simulink model "brushproportionelF"  (R2021a)
settings: Solver=ode45  StartTime=0.0  StopTime=2.0  RelTol=1e-3  EnableMultiTasking=on
libraries: spsIGBTDiodeLib x6, simulink x3, electricdrivelib x1, spsDCVoltageSourceLib x1, spspowerguiLib x1
settings Model: Creator=hp  LastModifiedBy=HP
settings SolverCC: AlgebraicLoopSolver=TrustRegion
settings DataIOCC: LimitDataPoints=on  SaveFormat=Array  ReturnWorkspaceOutputs=off
settings OptimizationCC: LifeSpan=inf
settings DebuggingCC: UnderspecifiedInitializationDetection=Classic  MergeDetectMultiDrivingBlocksExec=none  SolverPrmCheckMsg=warning  StateNameClashWarn=warning  SFUnexpectedBacktrackingDiag=warning  SFNoUnconditionalDefaultTransitionDiag=warning  SFExecutionAtInitializationDiag=none  SFMachineParentedDataDiag=warning  ArithmeticOperatorsInVariantConditions=warning
settings HardwareCC: ProdBitPerPointer=32  ProdBitPerSizeT=32  ProdBitPerPtrDiffT=32  ProdLargestAtomicFloat=None  ProdIntDivRoundTo=Undefined  ProdEndianess=Unspecified  ProdWordSize=32  ProdHWDeviceType=32-bit Generic
settings ModelReferenceCC: PropagateSignalLabelsOutOfModel=off
settings SFSimCC: SimUseLocalCustomCode=off  CustomCodeUndefinedFunction=UseInterfaceOnly
settings RTWCC: RTWUseLocalCustomCode=off
settings CodeAppCC: StateflowObjectComments=on
settings GRTTargetCC: TargetLangStandard=C89/C90 (ANSI)
settings ConfigComp: CovMetricSettings=dw  CovSaveCumulativeToWorkspaceVar=on  CovSaveSingleToWorkspaceVar=on  CovExternalEMLEnable=off
settings SimscapeCC: SimscapeNormalizeSystem=off

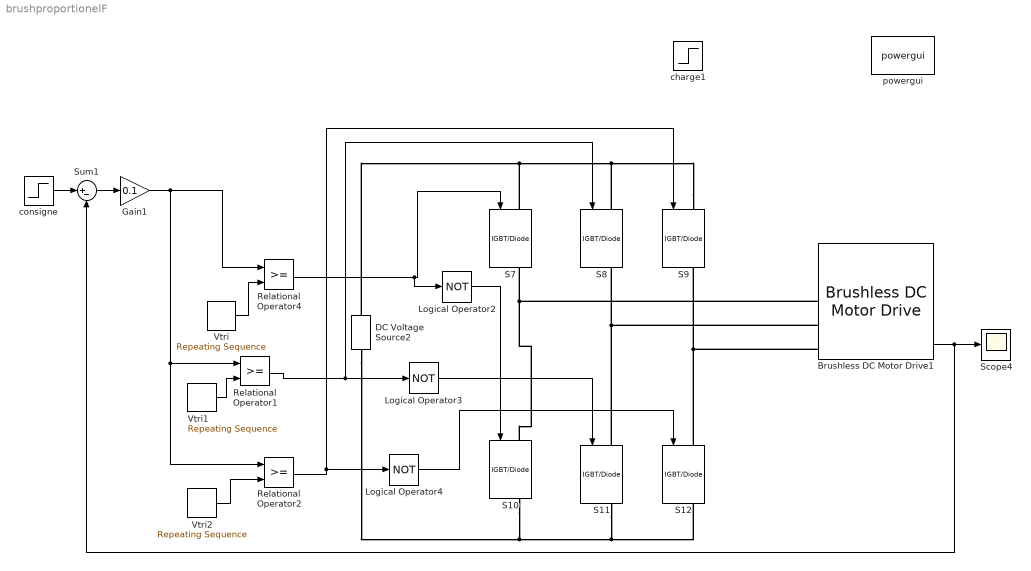
== system brushproportionelF ==
  Brushless DC Motor Drive1 : electricdrivelib/AC drives/Brushless DC Motor Drive  Rs=0.2  Lls=8.5e-3  Flat=120  MachineConstant=Flux linkage established by magnets (V.s)  FluxCst=0.175  VoltageCst=146.6077  TorqueCst=1.4  ia=0  ib=0  J=0.089  Friction=0.005  p=4  wm=0  thetam=0  Rsnb_rec=10e3  Csnb_rec=20e-9  Ron_rec=1e-3  Vf_rec=1.3  cap_bus=2000e-6  Rbrake=8  fbrake=4000  activationVoltage=320  shutdownVoltage=310  deviceType=MOSFET / Diodes  Ron_inv=1e-3  Vf_inv=0.8  Vfd_inv=0.8  Tf=1e-6  Tt=2e-6  Tf_GTO=10e-6  Tt_GTO=20e-6  Rsnb_inv=5000  Csnb_inv=1e-6  regulationType=Speed regulation  Acc=1000  Dec=-1000  kp_sc=5  ki_sc=100  fc_sc=100  Tsc=7*20e-6  Tmin=-17.8  Tmax=17.8  h=0.01  freq_max=20e3  Tvect=20e-6  zeta=0.99  Trd=0.13/5  K1=3000  K2=-49500  baseSampleTime=2e-06  outputBusMode=Multiple output buses  busLabels=off  sensorless=off  MechanicalLoad=Torque Tm  modelDetailLevel=Detailed  driveType=AC7  AverageValue=off
      settings: SourceProductBaseCode=PS
  DC Voltage Source2 : spsDCVoltageSourceLib/DC Voltage Source  Amplitude=240  Measurements=None
  Gain1 : Gain  Gain=0.1
  Logical Operator2 : Logic  Operator=NOT  AllPortsSameDT=off  OutDataTypeStr=boolean
  Logical Operator3 : Logic  Operator=NOT  AllPortsSameDT=off  OutDataTypeStr=boolean
  Logical Operator4 : Logic  Operator=NOT  AllPortsSameDT=off  OutDataTypeStr=boolean
  Relational Operator1 : RelationalOperator  OutDataTypeStr=boolean  RndMeth=Nearest
  Relational Operator2 : RelationalOperator  OutDataTypeStr=boolean  RndMeth=Nearest
  Relational Operator4 : RelationalOperator  OutDataTypeStr=boolean  RndMeth=Nearest
  S{7..12} (6 alike) : spsIGBTDiodeLib/IGBT//Diode  Ron=1e-3  Rs=1e5  Cs=inf  Measurements=on
  Scope4 : Scope
  Sum1 : Sum  Inputs=|+-
  Vtri : simulink/Sources/Repeating Sequence  rep_seq_t=[0 (1/2) 1]*0.001  rep_seq_y="[-1  1 -1] *240"
  Vtri1 : simulink/Sources/Repeating Sequence  rep_seq_t=[0 (1/6) 1]*0.001  rep_seq_y="[-1  1 -1] *240"
  Vtri2 : simulink/Sources/Repeating Sequence  rep_seq_t=[0 (1/3) 1]*0.001  rep_seq_y="[-1  1 -1] *240"
  charge1 : Step  Time=0.1  After=0.1  SampleTime=0
  consigne : Step  Time=0  After=150  SampleTime=0
  powergui : spspowerguiLib/powergui  Priority=1  SimulationMode=Discrete  SampleTime=1e-6  frequency=60  Iterations=50  frequencyindice=0  Pbase=100e6  ErrMax=1e-4  UnitsV=kV  UnitsW=MW  buscounter=0  FunctionMessages=off  echomessages=off  EnableUseOfTLC=off  CurrentSourceSwitches=off  DisableSnubberDevices=off  DisableRonSwitches=off  DisableVfSwitches=off  DisplayEquations=off  AutomaticDiscreteSolvers=off  SolverType=Tustin  Interpol=off  ExternalGateDelay=off  methode=off  Ts=0  x0status=blocks  SPID=off  SwTol=0  HookPort=off  NonlinearTolerance=1e-4  nMaxIteration=100  ContinueOnMaxIteration=off  RestoreLinks=warning  ResistiveCurrentMeasurement=off  Frange=[0:2:500]  Ylog=off  Xlog=on  ShowGrid=off  save=off  variable=ZData  structure=0  ZoomFFT=off  StartTime=0.0  cycles=1  DisplayStyle=1  fundamental=60  FreqAxis=off  MaxFrequency=1000  frequencyindicesteady=1  RmsSteady=1  display=off
  wires:
  Relational Operator4/1 -> Logical Operator2/1, S7/1
  Logical Operator2/1 -> S10/1
  Relational Operator1/1 -> S8/1, Logical Operator3/1
  Logical Operator3/1 -> S11/1
  Relational Operator2/1 -> Logical Operator4/1, S9/1
  Logical Operator4/1 -> S12/1
  Vtri1/1 -> Relational Operator1/2
  Gain1/1 -> Relational Operator2/1, Relational Operator1/1, Relational Operator4/1
  Vtri2/1 -> Relational Operator2/2
  Vtri/1 -> Relational Operator4/2
  consigne/1 -> Sum1/1
  Sum1/1 -> Gain1/1
  Brushless DC Motor Drive1/4 -> Sum1/2, Scope4/1
  connections:
  S9/RConn1 -- S12/LConn1 -- Brushless DC Motor Drive1/LConn3
  S12/RConn1 -- S11/RConn1 -- DC Voltage Source2/LConn1 -- S10/RConn1
  S9/LConn1 -- S8/LConn1 -- DC Voltage Source2/RConn1 -- S7/LConn1
  S7/RConn1 -- S10/LConn1 -- Brushless DC Motor Drive1/LConn1
  S8/RConn1 -- S11/LConn1 -- Brushless DC Motor Drive1/LConn2
